simulink model "SYSTEME_ZIGBEE_2017"  (R2016b)
settings: Solver=ode45  StartTime=0.0  StopTime=1E-3  RelTol=1e-3
libraries: dspsrcs4 x6, dsparch4 x5, simulink x2, simulink_extras x1, commsink2 x1, commrandsrc2 x1, commdigbbndcpm2 x1, dspsigops x1
settings Model: DisableUpgradeWarningsForVersion=R2015a  Creator=Yannis  LastModifiedBy=flori
settings DataIOCC: LimitDataPoints=on  SaveFormat=Array
settings OptimizationCC: BlockReduction=off  BooleanDataType=off  LifeSpan=inf
settings DebuggingCC: SaveWithParameterizedLinksMsg=none  UnderspecifiedInitializationDetection=Classic  MergeDetectMultiDrivingBlocksExec=none  SignalResolutionControl=TryResolveAllWithWarning  SFUnexpectedBacktrackingDiag=warning  SFNoUnconditionalDefaultTransitionDiag=warning  SFExecutionAtInitializationDiag=none
settings HardwareCC: ProdBitPerPointer=32  ProdBitPerSizeT=32  ProdBitPerPtrDiffT=32  ProdLargestAtomicFloat=None  ProdIntDivRoundTo=Undefined  ProdEndianess=Unspecified  ProdWordSize=32  ProdHWDeviceType=32-bit Generic  TargetBitPerPointer=64  TargetBitPerSizeT=64  TargetBitPerPtrDiffT=64  TargetLongLongMode=on  TargetIntDivRoundTo=Zero  TargetEndianess=LittleEndian  TargetWordSize=64  TargetHWDeviceType=MATLAB Host  ProdEqTarget=off
settings ModelReferenceCC: PropagateSignalLabelsOutOfModel=off
settings GRTTargetCC: TargetLangStandard=C89/C90 (ANSI)  GeneratePreprocessorConditionals=Disable all
settings ConfigComp: CovMetricSettings=dw  CovHtmlReporting=on  CovSaveCumulativeToWorkspaceVar=on  CovSaveSingleToWorkspaceVar=on  CovExternalEMLEnable=off

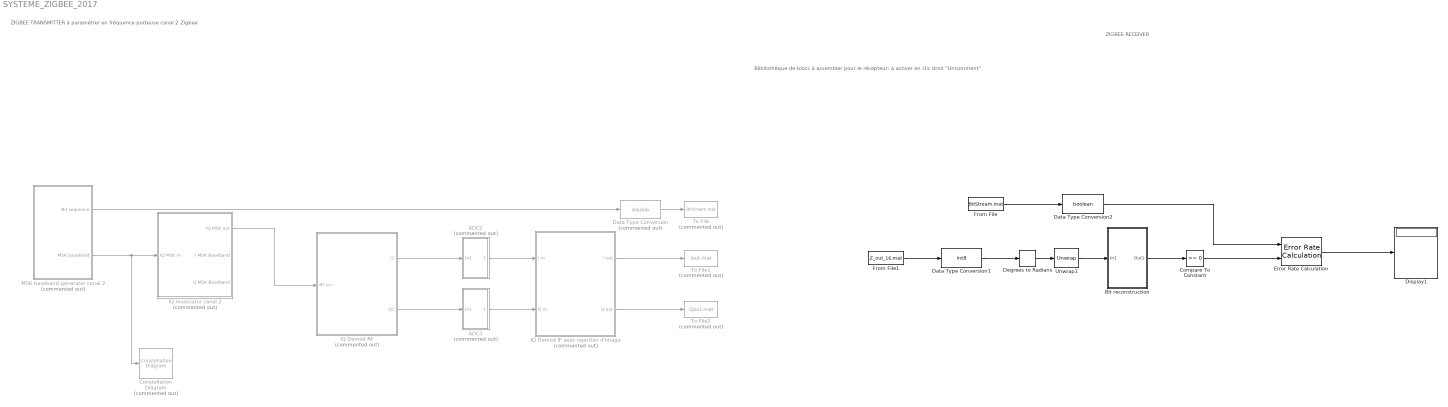
== system SYSTEME_ZIGBEE_2017 ==
  note: ZIGBEE RECEIVER
  note: ZIGBEE TRANSMITTER
      | à paramétrer en fréquence porteuse
      | canal 2  Zigbee
  note: Blibliothèque de blocs à assembler pour le récepteur: à activer en clic droit "Uncomment"
  ADC2 : Subsystem  Commented=on
  ADC3 : Subsystem  Commented=on
  Bit reconstruction : Subsystem
  Compare To Constant : simulink/Logic and Bit Operations/Compare To Constant  relop=>=  const=0  OutDataTypeStr=boolean
  Constellation Diagram : ConstellationDiagram  Commented=on
  Data Type Conversion : DataTypeConversion  Commented=on  OutDataTypeStr=double
  Data Type Conversion1 : DataTypeConversion  OutDataTypeStr=int8
  Data Type Conversion2 : DataTypeConversion  OutDataTypeStr=boolean
  Degrees to Radians : simulink_extras/Transformations/Degrees to Radians
  Display1 : Display
  Error Rate Calculation : commsink2/Error Rate Calculation  N=2  st_delay=1  cp_mode=Entire frame  subframe=[]  PMode=Port  WsName=ErrorVec  RsMode2=off  stop=off  numErr=100  maxBits=1e6
  From File : FromFile  FileName=BitStream.mat  OutDataTypeStr=fixdt('boolean', 'DataTypeOverride', 'Off')  SampleTime=1  ExtrapolationBeforeFirstDataPoint=Hold first value  InterpolationWithinTimeRange=Zero order hold  ExtrapolationAfterLastDataPoint=Hold last value
  From File1 : FromFile  FileName=Z_out_16.mat  OutDataTypeStr=int8  SampleTime=1  ExtrapolationBeforeFirstDataPoint=Hold first value  InterpolationWithinTimeRange=Zero order hold  ExtrapolationAfterLastDataPoint=Hold last value
  IQ Demod IF avec rejection d'image : Subsystem  Commented=on  TreatAsAtomicUnit=on
  IQ Demod RF : Subsystem  Commented=on  TreatAsAtomicUnit=on
  IQ modulator canal 2 : Subsystem  Commented=on
  MSK baseband generator canal 2 : Subsystem  Commented=on
  To File : ToFile  Commented=on  Filename=BitStream.mat  MatrixName=bit
  To File1 : ToFile  Commented=on  Filename=Iout.mat  MatrixName=iout
  To File2 : ToFile  Commented=on  Filename=Qout.mat  MatrixName=qout
  Unwrap1 : dspsigops/Unwrap  tol=pi  InputProcessing=Columns as channels (frame based)  running=off
  wires:
  MSK baseband generator canal 2/2(MSK baseband) -> IQ modulator canal 2/1(IQ MSK in), Constellation Diagram/1
  Error Rate Calculation/1 -> Display1/1
  MSK baseband generator canal 2/1(Bit sequence) -> Data Type Conversion/1
  IQ Demod RF/1(I1) -> ADC2/1(In1)
  ADC2/1(Out1) -> IQ Demod IF avec rejection d'image/1("I in ")
  IQ Demod RF/2("Q1 ") -> ADC3/1(In1)
  ADC3/1(Out1) -> IQ Demod IF avec rejection d'image/2("Q in ")
  IQ Demod IF avec rejection d'image/1(I out) -> To File1/1
  IQ Demod IF avec rejection d'image/2(Q out) -> To File2/1
  IQ modulator canal 2/1("IQ MSK out ") -> IQ Demod RF/1(RF in I)
  Data Type Conversion/1 -> To File/1
  From File1/1 -> Data Type Conversion1/1
  Data Type Conversion1/1 -> Degrees to Radians/1
  Degrees to Radians/1 -> Unwrap1/1
  Unwrap1/1 -> Bit reconstruction/1(In1)
  Bit reconstruction/1(Out1) -> Compare To Constant/1
  Compare To Constant/1 -> Error Rate Calculation/2
  From File/1 -> Data Type Conversion2/1
  Data Type Conversion2/1 -> Error Rate Calculation/1

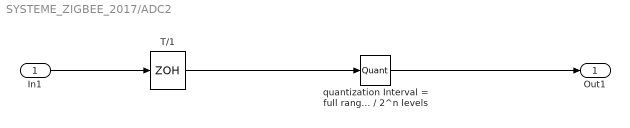
== system SYSTEME_ZIGBEE_2017/ADC2 ==
  In1 : Inport
  T/1 : ZeroOrderHold  SampleTime=1/(10e6)
  quantization Interval = full range (2Volts) / 2^n levels : Quantizer  QuantizationInterval=2/256  LinearizeAsGain=off  SampleTime=1/(10e6)
  Out1 : Outport
  wires:
  In1/1 -> T/1/1
  T/1/1 -> quantization Interval = full range (2Volts) / 2^n levels/1
  quantization Interval = full range (2Volts) / 2^n levels/1 -> Out1/1

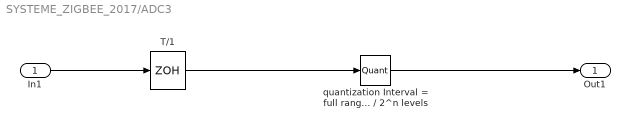
== system SYSTEME_ZIGBEE_2017/ADC3 ==
  In1 : Inport
  T/1 : ZeroOrderHold  SampleTime=1/(10e6)
  quantization Interval = full range (2Volts) / 2^n levels : Quantizer  QuantizationInterval=2/256  LinearizeAsGain=off  SampleTime=1/(10e6)
  Out1 : Outport
  wires:
  In1/1 -> T/1/1
  T/1/1 -> quantization Interval = full range (2Volts) / 2^n levels/1
  quantization Interval = full range (2Volts) / 2^n levels/1 -> Out1/1

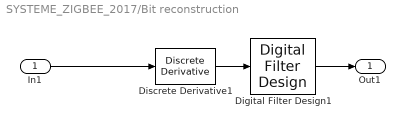
== system SYSTEME_ZIGBEE_2017/Bit reconstruction ==
  In1 : Inport
  Digital Filter Design1 : dsparch4/Digital Filter Design  mwdsp_browser_bugfix_var=off
  Discrete Derivative1 : simulink/Discrete/Discrete Derivative  gainval=1/(10e6)  ICPrevScaledInput=0.0  InputProcessing=Inherited  OutMin=[]  OutMax=[]  OutDataTypeStr=double  OutputDataTypeScalingMode=double  OutDataType=fixdt(1, 16)  OutScaling=2^-10  DoSatur=off
  Out1 : Outport
  wires:
  Discrete Derivative1/1 -> Digital Filter Design1/1
  Digital Filter Design1/1 -> Out1/1
  In1/1 -> Discrete Derivative1/1

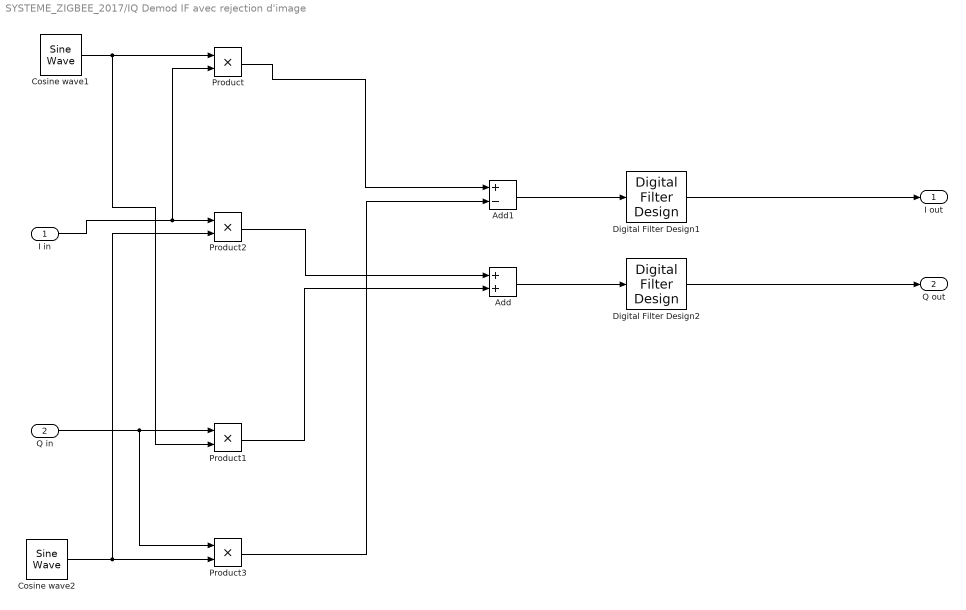
== system SYSTEME_ZIGBEE_2017/IQ Demod IF avec rejection d'image ==
  "I in " : Inport
  "Q in " : Inport  Port=2
  Add : Sum
  Add1 : Sum  Inputs=+-
  Cosine wave1 : dspsrcs4/Sine Wave  Amplitude=1  Frequency=2.5e6  Phase=pi/2  SampleMode=Discrete  OutComplex=Real  CompMethod=Trigonometric fcn  TableSize=Speed  SampleTime=1/(10e6)  SamplesPerFrame=1  ResetState=Restart at time zero  dataType=double  wordLen=16  udDataType=sfix(16)  fracBitsMode=Best precision  numFracBits=15  OutDataTypeStr=double  LastOutDataTypeStr=double
  Cosine wave2 : dspsrcs4/Sine Wave  Amplitude=1  Frequency=2.5e6  Phase=pi  SampleMode=Discrete  OutComplex=Real  CompMethod=Trigonometric fcn  TableSize=Speed  SampleTime=1/(10e6)  SamplesPerFrame=1  ResetState=Restart at time zero  dataType=double  wordLen=16  udDataType=sfix(16)  fracBitsMode=Best precision  numFracBits=15  OutDataTypeStr=double  LastOutDataTypeStr=double
  Digital Filter Design1 : dsparch4/Digital Filter Design  mwdsp_browser_bugfix_var=off
  Digital Filter Design2 : dsparch4/Digital Filter Design  mwdsp_browser_bugfix_var=off
  Product{,1..3} (4 alike) : Product
  I out : Outport
  Q out : Outport  Port=2
  wires:
  Digital Filter Design1/1 -> I out/1
  Digital Filter Design2/1 -> Q out/1
  Cosine wave2/1 -> Product2/2, Product3/2
  Product/1 -> Add1/1
  Add/1 -> Digital Filter Design2/1
  "I in "/1 -> Product/2, Product2/1
  "Q in "/1 -> Product3/1, Product1/1
  Cosine wave1/1 -> Product1/2, Product/1
  Product3/1 -> Add1/2
  Product1/1 -> Add/2
  Product2/1 -> Add/1
  Add1/1 -> Digital Filter Design1/1

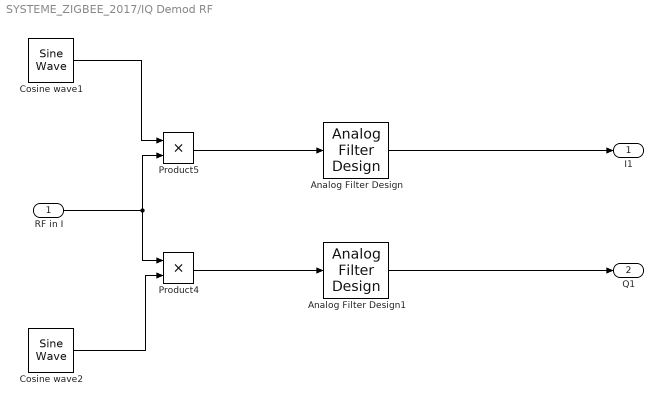
== system SYSTEME_ZIGBEE_2017/IQ Demod RF ==
  RF in I : Inport
  Analog Filter Design : dsparch4/Analog Filter Design  method=Butterworth  filttype=Lowpass  N=8  Wlo=31.4e6  Whi=80  Rp=2  Rs=40
  Analog Filter Design1 : dsparch4/Analog Filter Design  method=Butterworth  filttype=Lowpass  N=8  Wlo=31.4e6  Whi=80  Rp=2  Rs=40
  Cosine wave1 : dspsrcs4/Sine Wave  Amplitude=1  Frequency=2.4075e9  Phase=pi/2  SampleMode=Continuous  OutComplex=Real  CompMethod=Trigonometric fcn  TableSize=Speed  SampleTime=1/(10e6)  SamplesPerFrame=1  ResetState=Restart at time zero  dataType=double  wordLen=16  udDataType=sfix(16)  fracBitsMode=Best precision  numFracBits=15  OutDataTypeStr=double  LastOutDataTypeStr=double
  Cosine wave2 : dspsrcs4/Sine Wave  Amplitude=1  Frequency=2.4075e9  Phase=pi  SampleMode=Continuous  OutComplex=Real  CompMethod=Trigonometric fcn  TableSize=Speed  SampleTime=1/(10e6)  SamplesPerFrame=1  ResetState=Restart at time zero  dataType=double  wordLen=16  udDataType=sfix(16)  fracBitsMode=Best precision  numFracBits=15  OutDataTypeStr=double  LastOutDataTypeStr=double
  Product4 : Product  RndMeth=Zero
  Product5 : Product  RndMeth=Zero
  I1 : Outport
  "Q1 " : Outport  Port=2
  wires:
  RF in I/1 -> Product5/2, Product4/1
  Cosine wave2/1 -> Product4/2
  Cosine wave1/1 -> Product5/1
  Product5/1 -> Analog Filter Design/1
  Product4/1 -> Analog Filter Design1/1
  Analog Filter Design/1 -> I1/1
  Analog Filter Design1/1 -> "Q1 "/1

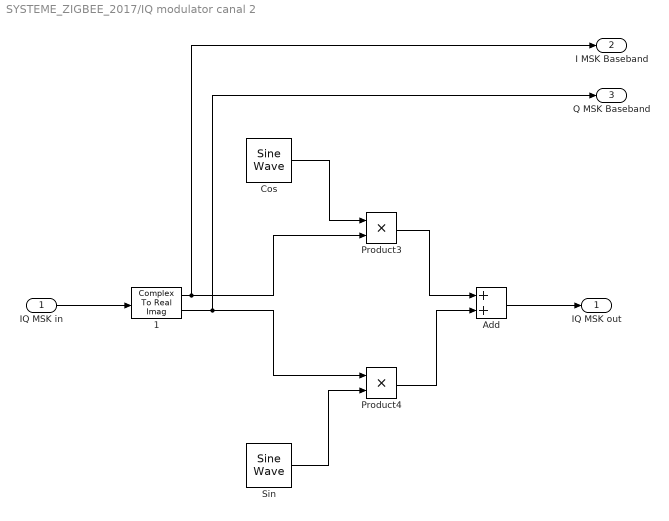
== system SYSTEME_ZIGBEE_2017/IQ modulator canal 2 ==
  IQ MSK in : Inport
  " 1" : ComplexToRealImag
  Add : Sum
  Cos : dspsrcs4/Sine Wave  Amplitude=1  Frequency=2.410e9  Phase=pi/2  SampleMode=Continuous  OutComplex=Real  CompMethod=Trigonometric fcn  TableSize=Speed  SampleTime=1/(8*2.4e9)  SamplesPerFrame=1  ResetState=Restart at time zero  dataType=double  wordLen=16  udDataType=sfix(16)  fracBitsMode=Best precision  numFracBits=15  OutDataTypeStr=double  LastOutDataTypeStr=double
  Product3 : Product  RndMeth=Zero
  Product4 : Product  RndMeth=Zero
  Sin : dspsrcs4/Sine Wave  Amplitude=1  Frequency=2.410e9  Phase=pi  SampleMode=Continuous  OutComplex=Real  CompMethod=Trigonometric fcn  TableSize=Speed  SampleTime=1/(4*2.4e9)  SamplesPerFrame=1  ResetState=Restart at time zero  dataType=double  wordLen=16  udDataType=sfix(16)  fracBitsMode=Best precision  numFracBits=15  OutDataTypeStr=double  LastOutDataTypeStr=double
  "IQ MSK out " : Outport
  I MSK Baseband : Outport  Port=2
  Q MSK Baseband : Outport  Port=3
  wires:
  Add/1 -> "IQ MSK out "/1
  Product4/1 -> Add/2
  " 1"/2 -> Product4/1, Q MSK Baseband/1
  " 1"/1 -> I MSK Baseband/1, Product3/2
  Sin/1 -> Product4/2
  Product3/1 -> Add/1
  Cos/1 -> Product3/1
  IQ MSK in/1 -> " 1"/1

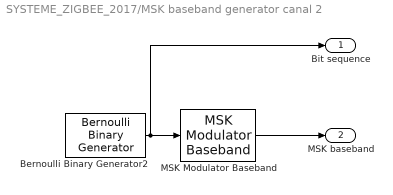
== system SYSTEME_ZIGBEE_2017/MSK baseband generator canal 2 ==
  Bernoulli Binary Generator2 : commrandsrc2/Bernoulli Binary Generator  P=0.5  seed=0  Ts=0.5e-6  frameBased=off  sampPerFrame=1  orient=off  outDataType=boolean
  MSK Modulator Baseband : commdigbbndcpm2/MSK Modulator Baseband  inputType=Bit  phaseOffset=0  samplesPerSymbol=20  RateOptions=Inherit from input (this choice will be removed - see release notes)  outDataType=double
  Bit sequence : Outport
  MSK baseband : Outport  Port=2
  wires:
  Bernoulli Binary Generator2/1 -> Bit sequence/1, MSK Modulator Baseband/1
  MSK Modulator Baseband/1 -> MSK baseband/1
